simulink model "nine_bus_main_model"  (R2024a)
settings: Solver=FixedStepAuto  StartTime=0.0  StopTime=0.5  FixedStep=2e-5  MaxStep=1e-4  RelTol=1e-3
libraries: spsThreePhaseBreakerLib x18, spsThreePhaseVIMeasurementLib x18, simulink x18, sdolib x9, spsSeriesRLCBranchLib x9, spsThreePhasePISectionLineLib x6, spsThreePhaseSourceLib x3, spsThreePhaseParallelRLCLoadLib x3, spsThreePhaseTransformerTwoWindingsLib x3, spsThreePhaseFaultLib x2, spspowerguiLib x1
settings Model: Creator=Vaibhav Chaudhary  LastModifiedBy=Vaibhav Chaudhary

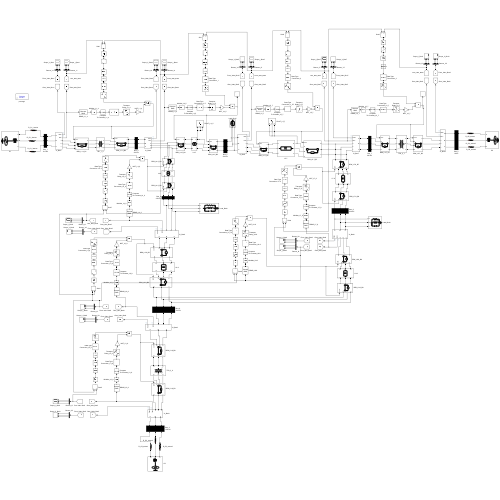
[thumbnail: Simulink's stored preview of the top-level diagram]
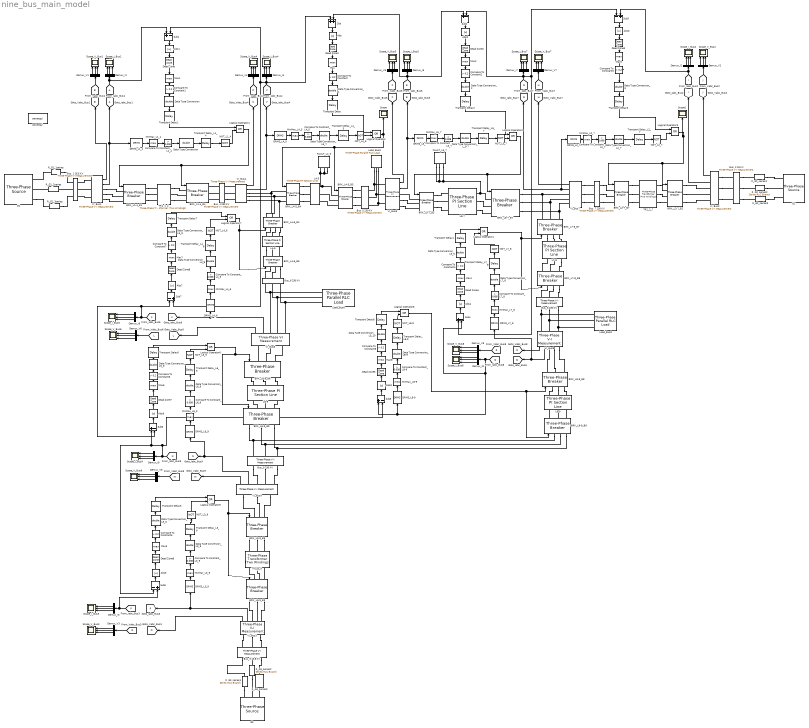
== system nine_bus_main_model ==
  Abs{,1..8} (9 alike) : Abs  SaturateOnIntegerOverflow=off
  "BRK_L1-4_B1 " : spsThreePhaseBreakerLib/Three-Phase Breaker  InitialState=closed  SwitchA=on  SwitchB=on  SwitchC=on  SwitchTimes="[1/60  5/60]"  External=on  BreakerResistance=0.01  SnubberResistance=1e6  SnubberCapacitance=inf  Measurements=None
  BRK_L1-4_B4 : spsThreePhaseBreakerLib/Three-Phase Breaker  InitialState=closed  SwitchA=on  SwitchB=on  SwitchC=on  SwitchTimes="[1/60  5/60]"  External=on  BreakerResistance=0.01  SnubberResistance=1e6  SnubberCapacitance=inf  Measurements=None
  "BRK_L2-7_B2 " : spsThreePhaseBreakerLib/Three-Phase Breaker  InitialState=closed  SwitchA=on  SwitchB=on  SwitchC=on  SwitchTimes="[1/60  5/60]"  External=on  BreakerResistance=0.01  SnubberResistance=1e6  SnubberCapacitance=inf  Measurements=None
  BRK_L2-7_B7 : spsThreePhaseBreakerLib/Three-Phase Breaker  InitialState=closed  SwitchA=on  SwitchB=on  SwitchC=on  SwitchTimes="[1/60  5/60]"  External=on  BreakerResistance=0.01  SnubberResistance=1e6  SnubberCapacitance=inf  Measurements=None
  "BRK_L3-9_B3 " : spsThreePhaseBreakerLib/Three-Phase Breaker  InitialState=closed  SwitchA=on  SwitchB=on  SwitchC=on  SwitchTimes="[1/60  5/60]"  External=on  BreakerResistance=0.01  SnubberResistance=1e6  SnubberCapacitance=inf  Measurements=None
  BRK_L3-9_B9 : spsThreePhaseBreakerLib/Three-Phase Breaker  InitialState=closed  SwitchA=on  SwitchB=on  SwitchC=on  SwitchTimes="[1/60  5/60]"  External=on  BreakerResistance=0.01  SnubberResistance=1e6  SnubberCapacitance=inf  Measurements=None
  BRK_L4-5_B4 : spsThreePhaseBreakerLib/Three-Phase Breaker  InitialState=closed  SwitchA=on  SwitchB=on  SwitchC=on  SwitchTimes="[1/60  5/60]"  External=on  BreakerResistance=0.01  SnubberResistance=1e6  SnubberCapacitance=inf  Measurements=None
  BRK_L4-5_B5 : spsThreePhaseBreakerLib/Three-Phase Breaker  InitialState=closed  SwitchA=on  SwitchB=on  SwitchC=on  SwitchTimes="[1/60  5/60]"  External=on  BreakerResistance=0.01  SnubberResistance=1e6  SnubberCapacitance=inf  Measurements=None
  BRK_L4-6_B4 : spsThreePhaseBreakerLib/Three-Phase Breaker  InitialState=closed  SwitchA=on  SwitchB=on  SwitchC=on  SwitchTimes="[1/60  5/60]"  External=on  BreakerResistance=0.01  SnubberResistance=1e6  SnubberCapacitance=inf  Measurements=None
  BRK_L4-6_B6 : spsThreePhaseBreakerLib/Three-Phase Breaker  InitialState=closed  SwitchA=on  SwitchB=on  SwitchC=on  SwitchTimes="[1/60  5/60]"  External=on  BreakerResistance=0.01  SnubberResistance=1e6  SnubberCapacitance=inf  Measurements=None
  BRK_L5-7_B5 : spsThreePhaseBreakerLib/Three-Phase Breaker  InitialState=closed  SwitchA=on  SwitchB=on  SwitchC=on  SwitchTimes="[1/60  5/60]"  External=on  BreakerResistance=0.01  SnubberResistance=1e6  SnubberCapacitance=inf  Measurements=None
  BRK_L5-7_B7 : spsThreePhaseBreakerLib/Three-Phase Breaker  InitialState=closed  SwitchA=on  SwitchB=on  SwitchC=on  SwitchTimes="[1/60  5/60]"  External=on  BreakerResistance=0.01  SnubberResistance=1e6  SnubberCapacitance=inf  Measurements=None
  BRK_L6-9_B6 : spsThreePhaseBreakerLib/Three-Phase Breaker  InitialState=closed  SwitchA=on  SwitchB=on  SwitchC=on  SwitchTimes="[1/60  5/60]"  External=on  BreakerResistance=0.01  SnubberResistance=1e6  SnubberCapacitance=inf  Measurements=None
  BRK_L6-9_B9 : spsThreePhaseBreakerLib/Three-Phase Breaker  InitialState=closed  SwitchA=on  SwitchB=on  SwitchC=on  SwitchTimes="[1/60  5/60]"  External=on  BreakerResistance=0.01  SnubberResistance=1e6  SnubberCapacitance=inf  Measurements=None
  BRK_L7-8_B7 : spsThreePhaseBreakerLib/Three-Phase Breaker  InitialState=closed  SwitchA=on  SwitchB=on  SwitchC=on  SwitchTimes="[1/60  5/60]"  External=on  BreakerResistance=0.01  SnubberResistance=1e6  SnubberCapacitance=inf  Measurements=None
  BRK_L7-8_B8 : spsThreePhaseBreakerLib/Three-Phase Breaker  InitialState=closed  SwitchA=on  SwitchB=on  SwitchC=on  SwitchTimes="[1/60  5/60]"  External=on  BreakerResistance=0.01  SnubberResistance=1e6  SnubberCapacitance=inf  Measurements=None
  BRK_L8-9_B8 : spsThreePhaseBreakerLib/Three-Phase Breaker  InitialState=closed  SwitchA=on  SwitchB=on  SwitchC=on  SwitchTimes="[1/60  5/60]"  External=on  BreakerResistance=0.01  SnubberResistance=1e6  SnubberCapacitance=inf  Measurements=None
  BRK_L8-9_B9 : spsThreePhaseBreakerLib/Three-Phase Breaker  InitialState=closed  SwitchA=on  SwitchB=on  SwitchC=on  SwitchTimes="[1/60  5/60]"  External=on  BreakerResistance=0.01  SnubberResistance=1e6  SnubberCapacitance=inf  Measurements=None
  Bus_1 16.5 KV : spsThreePhaseVIMeasurementLib/Three-Phase V-I Measurement  VoltageMeasurement=phase-to-phase  SetLabelV=on  LabelV=Vabc_B1  Vpu=on  VpuLL=off  CurrentMeasurement=yes  SetLabelI=on  LabelI=Iabc_B1  Ipu=on  Pbase=100e6  Vbase=16.5e3  OutputType=Complex  PhasorSimulation=off  PSBequivalent=0
  Bus_2 18 KV : spsThreePhaseVIMeasurementLib/Three-Phase V-I Measurement  VoltageMeasurement=phase-to-phase  SetLabelV=on  LabelV=Vabc_B2  Vpu=on  VpuLL=off  CurrentMeasurement=yes  SetLabelI=on  LabelI=Iabc_B2  Ipu=on  Pbase=100e6  Vbase=18e3  OutputType=Complex  PhasorSimulation=off  PSBequivalent=0
  Bus_3 13.8 KV : spsThreePhaseVIMeasurementLib/Three-Phase V-I Measurement  VoltageMeasurement=phase-to-phase  SetLabelV=on  LabelV=Vabc_B3  Vpu=on  VpuLL=off  CurrentMeasurement=yes  SetLabelI=on  LabelI=Iabc_B3  Ipu=on  Pbase=100e6  Vbase=13.8e3  OutputType=Complex  PhasorSimulation=off  PSBequivalent=0
  Bus_4 230 KV : spsThreePhaseVIMeasurementLib/Three-Phase V-I Measurement  VoltageMeasurement=phase-to-phase  SetLabelV=on  LabelV=Vabc_B4  Vpu=on  VpuLL=off  CurrentMeasurement=yes  SetLabelI=on  LabelI=Iabc_B4  Ipu=on  Pbase=100e6  Vbase=230e3  OutputType=Complex  PhasorSimulation=off  PSBequivalent=0
  Bus_5 230 KV : spsThreePhaseVIMeasurementLib/Three-Phase V-I Measurement  VoltageMeasurement=phase-to-phase  SetLabelV=on  LabelV=Vabc_B5  Vpu=on  VpuLL=off  CurrentMeasurement=yes  SetLabelI=on  LabelI=Iabc_B5  Ipu=on  Pbase=100e6  Vbase=230e3  OutputType=Complex  PhasorSimulation=off  PSBequivalent=0
  Bus_6 230 KV : spsThreePhaseVIMeasurementLib/Three-Phase V-I Measurement  VoltageMeasurement=phase-to-phase  SetLabelV=on  LabelV=Vabc_B6  Vpu=on  VpuLL=off  CurrentMeasurement=yes  SetLabelI=on  LabelI=Iabc_B6  Ipu=on  Pbase=100e6  Vbase=230e3  OutputType=Complex  PhasorSimulation=off  PSBequivalent=0
  Bus_7 230 KV : spsThreePhaseVIMeasurementLib/Three-Phase V-I Measurement  VoltageMeasurement=phase-to-phase  SetLabelV=on  LabelV=Vabc_B7  Vpu=on  VpuLL=off  CurrentMeasurement=yes  SetLabelI=on  LabelI=Iabc_B7  Ipu=on  Pbase=100e6  Vbase=230e3  OutputType=Complex  PhasorSimulation=off  PSBequivalent=0
  Bus_8 230 KV : spsThreePhaseVIMeasurementLib/Three-Phase V-I Measurement  VoltageMeasurement=phase-to-phase  SetLabelV=on  LabelV=Vabc_B8  Vpu=on  VpuLL=off  CurrentMeasurement=yes  SetLabelI=on  LabelI=Iabc_B8  Ipu=on  Pbase=100e6  Vbase=230e3  OutputType=Complex  PhasorSimulation=off  PSBequivalent=0
  Bus_9 230 KV : spsThreePhaseVIMeasurementLib/Three-Phase V-I Measurement  VoltageMeasurement=phase-to-phase  SetLabelV=on  LabelV=Vabc_B9  Vpu=on  VpuLL=off  CurrentMeasurement=yes  SetLabelI=on  LabelI=Iabc_B9  Ipu=on  Pbase=100e6  Vbase=230e3  OutputType=Complex  PhasorSimulation=off  PSBequivalent=0
  Compare To Constant{,1..8} (9 alike) : simulink/Logic and Bit Operations/Compare To Constant  relop=>  const=0.2  OutDataTypeStr=boolean
  Compare To Constant_L1_4 : simulink/Logic and Bit Operations/Compare To Constant  relop=>  const=0.008  OutDataTypeStr=boolean
  Compare To Constant_L2_7 : simulink/Logic and Bit Operations/Compare To Constant  relop=>  const=0.008  OutDataTypeStr=boolean
  Compare To Constant_L3_9 : simulink/Logic and Bit Operations/Compare To Constant  relop=>  const=0.008  OutDataTypeStr=boolean
  Compare To Constant_L4_5 : simulink/Logic and Bit Operations/Compare To Constant  relop=>  const=0.008  OutDataTypeStr=boolean
  Compare To Constant_L4_6 : simulink/Logic and Bit Operations/Compare To Constant  relop=>  const=0.008  OutDataTypeStr=boolean
  Compare To Constant_L5_7 : simulink/Logic and Bit Operations/Compare To Constant  relop=>  const=0.008  OutDataTypeStr=boolean
  Compare To Constant_L6_9 : simulink/Logic and Bit Operations/Compare To Constant  relop=>  const=0.008  OutDataTypeStr=boolean
  Compare To Constant_L7_8 : simulink/Logic and Bit Operations/Compare To Constant  relop=>  const=0.008  OutDataTypeStr=boolean
  Compare To Constant_L8-9 : simulink/Logic and Bit Operations/Compare To Constant  relop=>  const=0.008  OutDataTypeStr=boolean
  DRMS_L1_4 : sdolib/RMS Blocks/DRMS  Ts=1
  DRMS_L2_7 : sdolib/RMS Blocks/DRMS  Ts=1
  DRMS_L3_9 : sdolib/RMS Blocks/DRMS  Ts=1
  DRMS_L4_5 : sdolib/RMS Blocks/DRMS  Ts=1
  DRMS_L4_6 : sdolib/RMS Blocks/DRMS  Ts=1
  DRMS_L5_7 : sdolib/RMS Blocks/DRMS  Ts=1
  DRMS_L6_9 : sdolib/RMS Blocks/DRMS  Ts=1
  DRMS_L7_8 : sdolib/RMS Blocks/DRMS  Ts=1
  DRMS_L8-9 : sdolib/RMS Blocks/DRMS  Ts=1
  Data Type Conversion : DataTypeConversion  OutDataTypeStr=double  SaturateOnIntegerOverflow=off  RndMeth=Floor
  Data Type Conversion_1 : DataTypeConversion  OutDataTypeStr=double  SaturateOnIntegerOverflow=off  RndMeth=Floor
  Data Type Conversion_2 : DataTypeConversion  OutDataTypeStr=double  SaturateOnIntegerOverflow=off  RndMeth=Floor
  Data Type Conversion_3 : DataTypeConversion  OutDataTypeStr=double  SaturateOnIntegerOverflow=off  RndMeth=Floor
  Data Type Conversion_L5_{5..10} (6 alike) : DataTypeConversion  OutDataTypeStr=double  SaturateOnIntegerOverflow=off  RndMeth=Floor
  Data Type Conversion_L_5-7 : DataTypeConversion  OutDataTypeStr=double  SaturateOnIntegerOverflow=off  RndMeth=Floor
  Data Type Conversion_L2_7 : DataTypeConversion  OutDataTypeStr=double  SaturateOnIntegerOverflow=off  RndMeth=Floor
  Data Type Conversion_L3_9 : DataTypeConversion  OutDataTypeStr=double  SaturateOnIntegerOverflow=off  RndMeth=Floor
  Data Type Conversion_L4_6 : DataTypeConversion  OutDataTypeStr=double  SaturateOnIntegerOverflow=off  RndMeth=Floor
  Data Type Conversion_L6_9 : DataTypeConversion  OutDataTypeStr=double  SaturateOnIntegerOverflow=off  RndMeth=Floor
  Data Type Conversion_L7_8 : DataTypeConversion  OutDataTypeStr=double  SaturateOnIntegerOverflow=off  RndMeth=Floor
  Data Type Conversion_L8-9 : DataTypeConversion  OutDataTypeStr=double  SaturateOnIntegerOverflow=off  RndMeth=Floor
  Data Type Conversion : DataTypeConversion  OutDataTypeStr=double  SaturateOnIntegerOverflow=off  RndMeth=Floor
  Dead Zone{,2..8} (8 alike) : DeadZone  LowerValue=-0.01  UpperValue=0.01
  Dead Zone1 : DeadZone  LowerValue=0.01  UpperValue=inf
  Demux_I{1..9} (9 alike) : Demux  Outputs=3
  Demux_V{1..9} (9 alike) : Demux  Outputs=3
  FAULT_L4_5 : spsThreePhaseFaultLib/Three-Phase Fault  InitialStates=0  FaultA=on  FaultB=on  FaultC=on  GroundFault=on  SwitchTimes=[100 101]  External=off  SwitchStatus=NaN  FaultResistance=0.001  GroundResistance=0.001  SnubberResistance=1e6  SnubberCapacitance=inf  Measurements=None
  FAULT_L5_7 : spsThreePhaseFaultLib/Three-Phase Fault  InitialStates=0  FaultA=on  FaultB=on  FaultC=on  GroundFault=on  SwitchTimes=[0.05 0.1]  External=off  SwitchStatus=NaN  FaultResistance=0.001  GroundResistance=0.001  SnubberResistance=1e6  SnubberCapacitance=inf  Measurements=None
  From_Iabc_Bus1 : From  TagVisibility=global
  G1 : spsThreePhaseSourceLib/Three-Phase Source  InternalConnection=Yg  VoltagePhases=off  Voltage=16.5e3  PhaseAngle=0  Voltage_phases=[25e3 25e3 25e3]/sqrt(3)  PhaseAngles_phases=[0 -120 +120]  Frequency=50  NonIdealSource=on  SpecifyImpedance=off  Resistance=0  Inductance=0.1e-3  ShortCircuitLevel=100e6  BaseVoltage=16.5e3  XRratio=7  BusType=swing  Pref=10e3  Qref=0  Prefabc=[10e3, 10e3, 10e3]  Qrefabc=[0, 0, 0]  Qmin=-inf  Qmax=inf
  G2 : spsThreePhaseSourceLib/Three-Phase Source  InternalConnection=Yg  VoltagePhases=off  Voltage=18e3  PhaseAngle=0  Voltage_phases=[25e3 25e3 25e3]/sqrt(3)  PhaseAngles_phases=[0 -120 +120]  Frequency=50  NonIdealSource=on  SpecifyImpedance=off  Resistance=0  Inductance=0.15e-3  ShortCircuitLevel=100e6  BaseVoltage=18e3  XRratio=7  BusType=PV  Pref=163e3  Qref=0  Prefabc=[10e3, 10e3, 10e3]  Qrefabc=[0, 0, 0]  Qmin=-300e6  Qmax=300e6
  G3 : spsThreePhaseSourceLib/Three-Phase Source  InternalConnection=Yg  VoltagePhases=off  Voltage=13.8e3  PhaseAngle=0  Voltage_phases=[25e3 25e3 25e3]/sqrt(3)  PhaseAngles_phases=[0 -120 +120]  Frequency=50  NonIdealSource=on  SpecifyImpedance=off  Resistance=0  Inductance=0.2e-3  ShortCircuitLevel=100e6  BaseVoltage=13.8e3  XRratio=7  BusType=PV  Pref=85e3  Qref=0  Prefabc=[10e3, 10e3, 10e3]  Qrefabc=[0, 0, 0]  Qmin=-300e6  Qmax=300e6
  Goto_Iabc_Bus1 : Goto  TagVisibility=global
  L4-5 : spsThreePhasePISectionLineLib/Three-Phase PI Section Line  LConnTagsString=a|b|c  RConnTagsString=A|B|C  Length=100  Frequency=50  Resistances=[0.02 0.06]  Inductances=[1e-3 3e-3]  Capacitances=[2e-8 1e-8]
  L4-6 : spsThreePhasePISectionLineLib/Three-Phase PI Section Line  LConnTagsString=a|b|c  RConnTagsString=A|B|C  Length=100  Frequency=50  Resistances=[0.02 0.06]  Inductances=[1e-3 3e-3]  Capacitances=[2e-8 1e-8]
  L5-7 : spsThreePhasePISectionLineLib/Three-Phase PI Section Line  LConnTagsString=a|b|c  RConnTagsString=A|B|C  Length=100  Frequency=50  Resistances=[0.02 0.06]  Inductances=[1e-3 3e-3]  Capacitances=[2e-8 1e-8]
  L6-9 : spsThreePhasePISectionLineLib/Three-Phase PI Section Line  LConnTagsString=a|b|c  RConnTagsString=A|B|C  Length=100  Frequency=50  Resistances=[0.02 0.06]  Inductances=[1e-3 3e-3]  Capacitances=[2e-8 1e-8]
  L7-8 : spsThreePhasePISectionLineLib/Three-Phase PI Section Line  LConnTagsString=a|b|c  RConnTagsString=A|B|C  Length=100  Frequency=50  Resistances=[0.02 0.06]  Inductances=[1e-3 3e-3]  Capacitances=[2e-8 1e-8]
  L8-9 : spsThreePhasePISectionLineLib/Three-Phase PI Section Line  LConnTagsString=a|b|c  RConnTagsString=A|B|C  Length=100  Frequency=50  Resistances=[0.02 0.06]  Inductances=[1e-3 3e-3]  Capacitances=[2e-8 1e-8]
  Load_Bus5 : spsThreePhaseParallelRLCLoadLib/Three-Phase Parallel RLC Load  LConnTagsString=A|B|C  Configuration=Y (grounded)  NominalVoltage=230e3  Vabc=[1e3 1e3 1e3]  Vabcp=[1e3 1e3 1e3]  NominalFrequency=50  UnbalancedPower=off  ActivePower=125e6  InductivePower=50e6  CapacitivePower=50e6  Pabc=[10e3 9e3 11e3]  QLabc=[100 90 110]  QCabc=[100 90 110]  Pabcp=[10e3 9e3 11e3]  QLabcp=[100 90 110]  QCabcp=[100 90 110]  Measurements=None  LoadType=constant PQ
  Load_Bus6 : spsThreePhaseParallelRLCLoadLib/Three-Phase Parallel RLC Load  LConnTagsString=A|B|C  Configuration=Y (grounded)  NominalVoltage=230e3  Vabc=[1e3 1e3 1e3]  Vabcp=[1e3 1e3 1e3]  NominalFrequency=50  UnbalancedPower=off  ActivePower=90e6  InductivePower=30e6  CapacitivePower=30e6  Pabc=[10e3 9e3 11e3]  QLabc=[100 90 110]  QCabc=[100 90 110]  Pabcp=[10e3 9e3 11e3]  QLabcp=[100 90 110]  QCabcp=[100 90 110]  Measurements=None  LoadType=constant PQ
  Load_Bus8 : spsThreePhaseParallelRLCLoadLib/Three-Phase Parallel RLC Load  LConnTagsString=A|B|C  Configuration=Y (grounded)  NominalVoltage=230e3  Vabc=[1e3 1e3 1e3]  Vabcp=[1e3 1e3 1e3]  NominalFrequency=50  UnbalancedPower=off  ActivePower=100e6  InductivePower=35e6  CapacitivePower=35e6  Pabc=[10e3 9e3 11e3]  QLabc=[100 90 110]  QCabc=[100 90 110]  Pabcp=[10e3 9e3 11e3]  QLabcp=[100 90 110]  QCabcp=[100 90 110]  Measurements=None  LoadType=constant PQ
  Logical Operator{,1..8} (9 alike) : Logic  Operator=OR  AllPortsSameDT=off  OutDataTypeStr=boolean
  Max{,1..8} (9 alike) : MinMax  Function=max
  MinMax_L1_4 : MinMax  Function=max
  MinMax_L2_7 : MinMax  Function=max
  MinMax_L3_9 : MinMax  Function=max
  MinMax_L4_5 : MinMax  Function=max
  MinMax_L4_6 : MinMax  Function=max
  MinMax_L5_7 : MinMax  Function=max
  MinMax_L6_9 : MinMax  Function=max
  MinMax_L7_8 : MinMax  Function=max
  MinMax_L8-9 : MinMax  Function=max
  NOT_L1_4 : Logic  Operator=NOT  IconShape=distinctive  AllPortsSameDT=off  OutDataTypeStr=boolean
  NOT_L2_7 : Logic  Operator=NOT  IconShape=distinctive  AllPortsSameDT=off  OutDataTypeStr=boolean
  NOT_L3_9 : Logic  Operator=NOT  IconShape=distinctive  AllPortsSameDT=off  OutDataTypeStr=boolean
  NOT_L4_5 : Logic  Operator=NOT  IconShape=distinctive  AllPortsSameDT=off  OutDataTypeStr=boolean
  NOT_L4_6 : Logic  Operator=NOT  IconShape=distinctive  AllPortsSameDT=off  OutDataTypeStr=boolean
  NOT_L5_7 : Logic  Operator=NOT  IconShape=distinctive  AllPortsSameDT=off  OutDataTypeStr=boolean
  NOT_L6_9 : Logic  Operator=NOT  IconShape=distinctive  AllPortsSameDT=off  OutDataTypeStr=boolean
  NOT_L7_8 : Logic  Operator=NOT  IconShape=distinctive  AllPortsSameDT=off  OutDataTypeStr=boolean
  NOT_L8-9 : Logic  Operator=NOT  IconShape=distinctive  AllPortsSameDT=off  OutDataTypeStr=boolean
  R_G1_1series : spsSeriesRLCBranchLib/Series RLC Branch  LConnTagsString=__new0  RConnTagsString=__new0  BranchType=R  Resistance=0.01  Inductance=1e-3  SetiL0=off  InitialCurrent=0  Capacitance=1e-6  Setx0=off  InitialVoltage=0  Measurements=None
  R_G1_2series : spsSeriesRLCBranchLib/Series RLC Branch  LConnTagsString=__new0  RConnTagsString=__new0  BranchType=R  Resistance=0.01  Inductance=1e-3  SetiL0=off  InitialCurrent=0  Capacitance=1e-6  Setx0=off  InitialVoltage=0  Measurements=None
  R_G1_3series : spsSeriesRLCBranchLib/Series RLC Branch  LConnTagsString=__new0  RConnTagsString=__new0  BranchType=R  Resistance=0.01  Inductance=1e-3  SetiL0=off  InitialCurrent=0  Capacitance=1e-6  Setx0=off  InitialVoltage=0  Measurements=None
  R_G2_series1 : spsSeriesRLCBranchLib/Series RLC Branch  LConnTagsString=__new0  RConnTagsString=__new0  BranchType=R  Resistance=0.01  Inductance=1e-3  SetiL0=off  InitialCurrent=0  Capacitance=1e-6  Setx0=off  InitialVoltage=0  Measurements=None
  R_G2_series2 : spsSeriesRLCBranchLib/Series RLC Branch  LConnTagsString=__new0  RConnTagsString=__new0  BranchType=R  Resistance=0.01  Inductance=1e-3  SetiL0=off  InitialCurrent=0  Capacitance=1e-6  Setx0=off  InitialVoltage=0  Measurements=None
  R_G2_series3 : spsSeriesRLCBranchLib/Series RLC Branch  LConnTagsString=__new0  RConnTagsString=__new0  BranchType=R  Resistance=0.01  Inductance=1e-3  SetiL0=off  InitialCurrent=0  Capacitance=1e-6  Setx0=off  InitialVoltage=0  Measurements=None
  R_G3_series1 : spsSeriesRLCBranchLib/Series RLC Branch  LConnTagsString=__new0  RConnTagsString=__new0  BranchType=R  Resistance=0.01  Inductance=1e-3  SetiL0=off  InitialCurrent=0  Capacitance=1e-6  Setx0=off  InitialVoltage=0  Measurements=None
  R_G3_series2 : spsSeriesRLCBranchLib/Series RLC Branch  LConnTagsString=__new0  RConnTagsString=__new0  BranchType=R  Resistance=0.01  Inductance=1e-3  SetiL0=off  InitialCurrent=0  Capacitance=1e-6  Setx0=off  InitialVoltage=0  Measurements=None
  R_G3_series3 : spsSeriesRLCBranchLib/Series RLC Branch  LConnTagsString=__new0  RConnTagsString=__new0  BranchType=R  Resistance=0.01  Inductance=1e-3  SetiL0=off  InitialCurrent=0  Capacitance=1e-6  Setx0=off  InitialVoltage=0  Measurements=None
  Scope : Scope
  Scope1 : Scope
  Scope_I_Bus{1..9} (9 alike) : Scope  NumInputPorts=3
  Scope_V_Bus{1..9} (9 alike) : Scope  NumInputPorts=3
  Sub : Sum
  Sub{1..8} (8 alike) : Sum  Inputs=+-
  TR1_1_4 : spsThreePhaseTransformerTwoWindingsLib/Three-Phase Transformer (Two Windings)  Winding1Connection=Yg  Winding2Connection=Yg  CoreType=Three single-phase transformers  SetSaturation=off  Hysteresis=off  DataFile='hysteresis'  SetInitialFlux=off  Measurements=None  UNITS=pu  NominalPower=[ 100e6 , 50 ]  Winding1=[ 16.5e3 , 0.002 , 0.08 ]  Winding2=[ 230e3 , 0.002 , 0.08 ]  Rm=0.002  Lm=0.08  L0=0.5  Saturation=[ 0,0 ; 0.0024,1.2 ; 1.0,1.52 ]  InitialFluxes=[ 0.8 , -0.8 , 0.7 ]  BreakLoop=off  DiscreteSolver=Trapezoidal iterative  DataType=off  TransfoNumber=1
  TR2_2_7 : spsThreePhaseTransformerTwoWindingsLib/Three-Phase Transformer (Two Windings)  Winding1Connection=Yg  Winding2Connection=Yg  CoreType=Three single-phase transformers  SetSaturation=off  Hysteresis=off  DataFile='hysteresis'  SetInitialFlux=off  Measurements=None  UNITS=pu  NominalPower=[ 100e6 , 50]  Winding1=[ 18e3 , 0.002 , 0.08 ]  Winding2=[ 23e3 , 0.002 , 0.08 ]  Rm=0.002  Lm=0.08  L0=0.5  Saturation=[ 0,0 ; 0.0024,1.2 ; 1.0,1.52 ]  InitialFluxes=[ 0.8 , -0.8 , 0.7 ]  BreakLoop=off  DiscreteSolver=Trapezoidal iterative  DataType=off  TransfoNumber=1
  TR3_3_9 : spsThreePhaseTransformerTwoWindingsLib/Three-Phase Transformer (Two Windings)  Winding1Connection=Yg  Winding2Connection=Yg  CoreType=Three single-phase transformers  SetSaturation=off  Hysteresis=off  DataFile='hysteresis'  SetInitialFlux=off  Measurements=None  UNITS=pu  NominalPower=[ 100e6 , 50 ]  Winding1=[ 16.5e3 , 0.002 , 0.08 ]  Winding2=[ 230e3 , 0.002 , 0.08 ]  Rm=0.002  Lm=0.08  L0=0.5  Saturation=[ 0,0 ; 0.0024,1.2 ; 1.0,1.52 ]  InitialFluxes=[ 0.8 , -0.8 , 0.7 ]  BreakLoop=off  DiscreteSolver=Trapezoidal iterative  DataType=off  TransfoNumber=1
  Transport Delay{,1..8} (9 alike) : TransportDelay  DelayTime=0.005
  Transport Delay_L1_4 : TransportDelay  DelayTime=0.02
  Transport Delay_L2_7 : TransportDelay  DelayTime=0.02
  Transport Delay_L3_9 : TransportDelay  DelayTime=0.02
  Transport Delay_L4_5 : TransportDelay  DelayTime=0.02
  Transport Delay_L4_6 : TransportDelay  DelayTime=0.02
  Transport Delay_L5_7 : TransportDelay  DelayTime=0.02
  Transport Delay_L6_9 : TransportDelay  DelayTime=0.02
  Transport Delay_L7_8 : TransportDelay  DelayTime=0.02
  Transport Delay_L8-9 : TransportDelay  DelayTime=0.02
  VI_Bus1 : spsThreePhaseVIMeasurementLib/Three-Phase V-I Measurement  VoltageMeasurement=phase-to-phase  SetLabelV=off  LabelV=Vabc  Vpu=off  VpuLL=on  CurrentMeasurement=yes  SetLabelI=off  LabelI=Iabc  Ipu=on  Pbase=100e6  Vbase=16.5e3  OutputType=Complex  PhasorSimulation=off  PSBequivalent=0
  VI_Bus2 : spsThreePhaseVIMeasurementLib/Three-Phase V-I Measurement  VoltageMeasurement=phase-to-phase  SetLabelV=off  LabelV=Vabc  Vpu=off  VpuLL=on  CurrentMeasurement=yes  SetLabelI=off  LabelI=Iabc  Ipu=on  Pbase=100e6  Vbase=18e3  OutputType=Complex  PhasorSimulation=off  PSBequivalent=0
  VI_Bus3 : spsThreePhaseVIMeasurementLib/Three-Phase V-I Measurement  VoltageMeasurement=phase-to-phase  SetLabelV=off  LabelV=Vabc  Vpu=on  VpuLL=off  CurrentMeasurement=yes  SetLabelI=off  LabelI=Iabc  Ipu=on  Pbase=100e6  Vbase=13.8e3  OutputType=Complex  PhasorSimulation=off  PSBequivalent=0
  VI_Bus{4..6,9} (4 alike) : spsThreePhaseVIMeasurementLib/Three-Phase V-I Measurement  VoltageMeasurement=phase-to-phase  SetLabelV=off  LabelV=Vabc  Vpu=off  VpuLL=on  CurrentMeasurement=yes  SetLabelI=off  LabelI=Iabc  Ipu=on  Pbase=100e6  Vbase=250e3  OutputType=Complex  PhasorSimulation=off  PSBequivalent=0
  VI_Bus7 : spsThreePhaseVIMeasurementLib/Three-Phase V-I Measurement  VoltageMeasurement=phase-to-phase  SetLabelV=off  LabelV=Vabc  Vpu=off  VpuLL=off  CurrentMeasurement=yes  SetLabelI=off  LabelI=Iabc  Ipu=on  Pbase=100e6  Vbase=250e3  OutputType=Complex  PhasorSimulation=off  PSBequivalent=0
  VI_Bus8 : spsThreePhaseVIMeasurementLib/Three-Phase V-I Measurement  VoltageMeasurement=phase-to-phase  SetLabelV=off  LabelV=Vabc  Vpu=off  VpuLL=off  CurrentMeasurement=yes  SetLabelI=off  LabelI=Iabc  Ipu=on  Pbase=100e6  Vbase=250e3  OutputType=Complex  PhasorSimulation=off  PSBequivalent=0
  powergui : spspowerguiLib/powergui  Priority=1  SimulationMode=Discrete  SampleTime=2e-5  frequency=60  Iterations=50  frequencyindice=0  Pbase=100e6  ErrMax=1e-4  UnitsV=kV  UnitsW=MW  buscounter=0  FunctionMessages=off  echomessages=off  EnableUseOfTLC=off  CurrentSourceSwitches=off  DisableSnubberDevices=off  DisableRonSwitches=off  DisableVfSwitches=off  DisplayEquations=off  AutomaticDiscreteSolvers=off  SolverType=Tustin/Backward Euler (TBE)  Interpol=off  ExternalGateDelay=off  methode=off  Ts=100  x0status=blocks  SPID=on  SwTol=0  HookPort=off  NonlinearTolerance=1e-4  nMaxIteration=100  ContinueOnMaxIteration=off  RestoreLinks=warning  ResistiveCurrentMeasurement=off  Frange=[0:2:500]  Ylog=off  Xlog=on  ShowGrid=off  save=off  variable=ZData  structure=0  ZoomFFT=off  StartTime=0.0  cycles=1  DisplayStyle=1  fundamental=60  FreqAxis=off  MaxFrequency=1000  frequencyindicesteady=1  RmsSteady=1  display=off
  tag scope: B=global, C=global, E=global, F=global, G=global, H=global, I=global, J=global, K=global, L=global, M=global, N=global, O=global, P=global, Q=global, R=global, V=global
  wires:
  Demux_V1/1 -> Scope_V_Bus1/1
  Demux_I1/1 -> Scope_I_Bus1/1
  Demux_I1/2 -> Scope_I_Bus1/2
  Demux_I1/3 -> Scope_I_Bus1/3
  VI_Bus1/1 -> [B]
  Demux_V4/2 -> Scope_V_Bus4/2
  VI_Bus4/1 -> [C]
  Demux_V4/3 -> Scope_V_Bus4/3
  [C] -> Demux_V4/1
  Demux_V4/1 -> Scope_V_Bus4/1
  VI_Bus5/1 -> [F]
  Demux_I5/2 -> Scope_I_Bus5/2
  Demux_V5/3 -> Scope_V_Bus5/3
  Demux_I5/3 -> Scope_I_Bus5/3
  Demux_V5/1 -> Scope_V_Bus5/1
  Demux_V5/2 -> Scope_V_Bus5/2
  Demux_I5/1 -> Scope_I_Bus5/1
  [E] -> Demux_I5/1, Sub2/1, Sub/2
  VI_Bus7/1 -> [H]
  Demux_V7/3 -> Scope_V_Bus7/3
  Demux_I7/3 -> Scope_I_Bus7/3
  Demux_I7/2 -> Scope_I_Bus7/2
  Demux_I7/1 -> Scope_I_Bus7/1
  Demux_V7/1 -> Scope_V_Bus7/1
  [H] -> Demux_V7/1
  Demux_V7/2 -> Scope_V_Bus7/2
  VI_Bus2/2 -> [I]
  Demux_V2/1 -> Scope_V_Bus2/1
  Demux_I2/1 -> Scope_I_Bus2/1
  Demux_V2/2 -> Scope_V_Bus2/2
  [J] -> Demux_V2/1
  Demux_I2/2 -> Scope_I_Bus2/2
  VI_Bus2/1 -> [J]
  Demux_V2/3 -> Scope_V_Bus2/3
  Demux_I2/3 -> Scope_I_Bus2/3
  [K] -> Sub6/2, Sub7/2, Demux_I6/1
  Demux_I6/1 -> Scope_I_Bus6/1
  Demux_V6/2 -> Scope_V_Bus6/2
  VI_Bus6/1 -> [L]
  Demux_I6/3 -> Scope_I_Bus6/3
  Demux_V6/3 -> Scope_V_Bus6/3
  [L] -> Demux_V6/1
  Demux_V6/1 -> Scope_V_Bus6/1
  Demux_I6/2 -> Scope_I_Bus6/2
  [M] -> Demux_V9/1
  Demux_I9/1 -> Scope_I_Bus9/1
  Demux_I9/2 -> Scope_I_Bus9/2
  Demux_V9/2 -> Scope_V_Bus9/2
  VI_Bus9/2 -> DRMS_L6_9/1, [N]
  Demux_V9/3 -> Scope_V_Bus9/3
  Demux_I9/3 -> Scope_I_Bus9/3
  Demux_V9/1 -> Scope_V_Bus9/1
  VI_Bus9/1 -> [M]
  [O] -> Demux_V3/1
  [P] -> Sub5/1, Demux_I3/1
  Demux_I3/1 -> Scope_I_Bus3/1
  Demux_I3/2 -> Scope_I_Bus3/2
  Demux_V3/2 -> Scope_V_Bus3/2
  VI_Bus3/2 -> [P], DRMS_L3_9/1
  Demux_V3/3 -> Scope_V_Bus3/3
  Demux_I3/3 -> Scope_I_Bus3/3
  Demux_V3/1 -> Scope_V_Bus3/1
  VI_Bus3/1 -> [O]
  [R] -> Demux_V8/1
  [Q] -> Demux_I8/1, Sub4/2, Sub8/1, DRMS_L8-9/1
  Demux_I8/1 -> Scope_I_Bus8/1
  Demux_I8/2 -> Scope_I_Bus8/2
  Demux_V8/2 -> Scope_V_Bus8/2
  VI_Bus8/2 -> DRMS_L7_8/1, [Q]
  Demux_V8/3 -> Scope_V_Bus8/3
  Demux_I8/3 -> Scope_I_Bus8/3
  Demux_V8/1 -> Scope_V_Bus8/1
  VI_Bus8/1 -> [R]
  Transport Delay_L6_9/1 -> NOT_L6_9/1
  Demux_I4/1 -> Scope_I_Bus4/1
  Demux_I4/3 -> Scope_I_Bus4/3
  Demux_I4/2 -> Scope_I_Bus4/2
  Transport Delay_L5_7/1 -> NOT_L5_7/1
  Transport Delay_L2_7/1 -> NOT_L2_7/1
  Transport Delay_L4_6/1 -> NOT_L4_6/1
  VI_Bus6/2 -> [K], DRMS_L4_6/1
  DRMS_L1_4/1 -> MinMax_L1_4/1
  MinMax_L1_4/1 -> Compare To Constant_L1_4/1
  Transport Delay_L1_4/1 -> NOT_L1_4/1
  DRMS_L4_5/1 -> MinMax_L4_5/1
  MinMax_L4_5/1 -> Compare To Constant_L4_5/1
  Compare To Constant_L1_4/1 -> Data Type Conversion/1
  Data Type Conversion/1 -> Transport Delay_L1_4/1
  Compare To Constant_L4_5/1 -> Data Type Conversion_L5_7/1
  Data Type Conversion_L5_7/1 -> Transport Delay_L4_5/1
  VI_Bus5/2 -> [E], DRMS_L5_7/1
  MinMax_L5_7/1 -> Compare To Constant_L5_7/1
  Data Type Conversion_L_5-7/1 -> Transport Delay_L5_7/1
  Compare To Constant_L5_7/1 -> Data Type Conversion_L_5-7/1
  DRMS_L5_7/1 -> MinMax_L5_7/1
  Data Type Conversion_L2_7/1 -> Transport Delay_L2_7/1
  Compare To Constant_L2_7/1 -> Data Type Conversion_L2_7/1
  DRMS_L2_7/1 -> MinMax_L2_7/1
  VI_Bus7/2 -> [G], DRMS_L2_7/1
  MinMax_L2_7/1 -> Compare To Constant_L2_7/1
  Data Type Conversion_L7_8/1 -> Transport Delay_L7_8/1
  MinMax_L7_8/1 -> Compare To Constant_L7_8/1
  DRMS_L7_8/1 -> MinMax_L7_8/1
  Compare To Constant_L7_8/1 -> Data Type Conversion_L7_8/1
  Transport Delay_L7_8/1 -> NOT_L7_8/1
  MinMax_L3_9/1 -> Compare To Constant_L3_9/1
  DRMS_L3_9/1 -> MinMax_L3_9/1
  Compare To Constant_L3_9/1 -> Data Type Conversion_L3_9/1
  Data Type Conversion_L3_9/1 -> Transport Delay_L3_9/1
  Transport Delay_L3_9/1 -> NOT_L3_9/1
  MinMax_L6_9/1 -> Compare To Constant_L6_9/1
  DRMS_L6_9/1 -> MinMax_L6_9/1
  Compare To Constant_L6_9/1 -> Data Type Conversion_L6_9/1
  Data Type Conversion_L6_9/1 -> Transport Delay_L6_9/1
  Compare To Constant_L4_6/1 -> Data Type Conversion_L4_6/1
  MinMax_L4_6/1 -> Compare To Constant_L4_6/1
  DRMS_L4_6/1 -> MinMax_L4_6/1
  Data Type Conversion_L4_6/1 -> Transport Delay_L4_6/1
  Sub/1 -> Abs/1
  Abs/1 -> Dead Zone1/1
  [F] -> Demux_V5/1
  Max/1 -> Compare To Constant/1
  Compare To Constant/1 -> Data Type Conversion_1/1
  Data Type Conversion_1/1 -> Transport Delay/1
  Transport Delay/1 -> Logical Operator/1
  Data Type Conversion/1 -> Transport Delay1/1
  Abs1/1 -> Dead Zone/1
  Compare To Constant1/1 -> Data Type Conversion/1
  Sub1/1 -> Abs1/1
  Max1/1 -> Compare To Constant1/1
  Transport Delay1/1 -> Logical Operator1/1
  VI_Bus1/2 -> Goto_Iabc_Bus1/1, DRMS_L1_4/1
  NOT_L1_4/1 -> Logical Operator1/2
  Logical Operator1/1 -> "BRK_L1-4_B1 "/1, BRK_L1-4_B4/1
  Data Type Conversion_2/1 -> Transport Delay2/1
  Transport Delay2/1 -> Logical Operator2/1
  Compare To Constant2/1 -> Data Type Conversion_2/1
  Max2/1 -> Compare To Constant2/1
  NOT_L5_7/1 -> Logical Operator2/2
  Logical Operator2/1 -> BRK_L5-7_B5/1, BRK_L5-7_B7/1
  NOT_L2_7/1 -> Logical Operator3/2
  Logical Operator3/1 -> Scope1/1, "BRK_L2-7_B2 "/1, BRK_L2-7_B7/1
  Data Type Conversion_3/1 -> Transport Delay3/1
  Abs3/1 -> Dead Zone3/1
  Compare To Constant3/1 -> Data Type Conversion_3/1
  Sub3/1 -> Abs3/1
  Max3/1 -> Compare To Constant3/1
  [G] -> Sub3/2, Sub4/1, Sub2/2, Demux_I7/1
  Data Type Conversion_L5_5/1 -> Transport Delay4/1
  Compare To Constant4/1 -> Data Type Conversion_L5_5/1
  Sub4/1 -> Abs4/1
  Max4/1 -> Compare To Constant4/1
  Transport Delay3/1 -> Logical Operator3/1
  Transport Delay4/1 -> Logical Operator4/1
  NOT_L7_8/1 -> Logical Operator4/2
  Logical Operator4/1 -> BRK_L7-8_B8/1, BRK_L7-8_B7/1
  Sub5/1 -> Abs5/1
  Compare To Constant5/1 -> Data Type Conversion_L5_6/1
  Data Type Conversion_L5_6/1 -> Transport Delay5/1
  Abs5/1 -> Dead Zone6/1
  Max5/1 -> Compare To Constant5/1
  NOT_L3_9/1 -> Logical Operator5/2
  Transport Delay5/1 -> Logical Operator5/1
  Logical Operator5/1 -> "BRK_L3-9_B3 "/1, BRK_L3-9_B9/1
  NOT_L6_9/1 -> Logical Operator6/2
  Logical Operator6/1 -> BRK_L6-9_B9/1, BRK_L6-9_B6/1
  Sub6/1 -> Abs6/1
  Compare To Constant6/1 -> Data Type Conversion_L5_8/1
  Data Type Conversion_L5_8/1 -> Transport Delay6/1
  Max6/1 -> Compare To Constant6/1
  Transport Delay6/1 -> Logical Operator6/1
  Max7/1 -> Compare To Constant7/1
  Data Type Conversion_L5_9/1 -> Transport Delay7/1
  Sub7/1 -> Abs7/1
  Compare To Constant7/1 -> Data Type Conversion_L5_9/1
  Transport Delay7/1 -> Logical Operator7/1
  Abs7/1 -> Dead Zone8/1
  NOT_L4_6/1 -> Logical Operator7/2
  Logical Operator7/1 -> BRK_L4-6_B6/1, BRK_L4-6_B4/1
  NOT_L8-9/1 -> Logical Operator8/2
  Transport Delay8/1 -> Logical Operator8/1
  Logical Operator8/1 -> BRK_L8-9_B8/1, BRK_L8-9_B9/1
  Compare To Constant8/1 -> Data Type Conversion_L5_10/1
  Data Type Conversion_L5_10/1 -> Transport Delay8/1
  Abs8/1 -> Dead Zone5/1
  Max8/1 -> Compare To Constant8/1
  Transport Delay_L8-9/1 -> NOT_L8-9/1
  MinMax_L8-9/1 -> Compare To Constant_L8-9/1
  Sub8/1 -> Abs8/1
  DRMS_L8-9/1 -> MinMax_L8-9/1
  Compare To Constant_L8-9/1 -> Data Type Conversion_L8-9/1
  Data Type Conversion_L8-9/1 -> Transport Delay_L8-9/1
  Dead Zone/1 -> Max1/1
  Dead Zone1/1 -> Max/1
  Dead Zone2/1 -> Max2/1
  Sub2/1 -> Abs2/1
  Dead Zone3/1 -> Max3/1
  Dead Zone4/1 -> Max4/1
  Dead Zone5/1 -> Max8/1
  Dead Zone6/1 -> Max5/1
  Dead Zone7/1 -> Max6/1
  Dead Zone8/1 -> Max7/1
  Logical Operator/1 -> BRK_L4-5_B4/1, BRK_L4-5_B5/1, Scope/1
  Transport Delay_L4_5/1 -> NOT_L4_5/1
  NOT_L4_5/1 -> Logical Operator/2
  VI_Bus4/2 -> DRMS_L4_5/1, [V]
  [B] -> Demux_V1/1
  From_Iabc_Bus1/1 -> Sub1/1, Demux_I1/1
  Abs2/1 -> Dead Zone2/1
  [I] -> Sub3/1, Demux_I2/1
  Abs4/1 -> Dead Zone4/1
  [N] -> Sub8/2, Sub5/2, Sub6/1, Demux_I9/1
  Abs6/1 -> Dead Zone7/1
  [V] -> Sub/1, Sub1/2, Sub7/1, Demux_I4/1
  Demux_V1/3 -> Scope_V_Bus1/3
  Demux_V1/2 -> Scope_V_Bus1/2
  connections:
  VI_Bus1/LConn3 -- Bus_1 16.5 KV/LConn3
  VI_Bus1/LConn2 -- Bus_1 16.5 KV/LConn2
  VI_Bus1/LConn1 -- Bus_1 16.5 KV/LConn1
  VI_Bus5/LConn3 -- Bus_5 230 KV/LConn3 -- Load_Bus5/LConn3
  VI_Bus5/LConn2 -- Bus_5 230 KV/LConn2 -- Load_Bus5/LConn2
  VI_Bus5/LConn1 -- Bus_5 230 KV/LConn1 -- Load_Bus5/LConn1
  VI_Bus2/LConn2 -- Bus_2 18 KV/LConn2
  VI_Bus2/LConn1 -- Bus_2 18 KV/LConn1
  VI_Bus2/LConn3 -- Bus_2 18 KV/LConn3
  VI_Bus7/LConn1 -- Bus_7 230 KV/LConn1
  VI_Bus7/LConn2 -- Bus_7 230 KV/LConn2
  VI_Bus7/LConn3 -- Bus_7 230 KV/LConn3
  Bus_8 230 KV/LConn3 -- VI_Bus8/LConn3 -- Load_Bus8/LConn3
  Bus_8 230 KV/LConn2 -- VI_Bus8/LConn2 -- Load_Bus8/LConn2
  Bus_8 230 KV/LConn1 -- VI_Bus8/LConn1 -- Load_Bus8/LConn1
  VI_Bus3/LConn1 -- Bus_3 13.8 KV/LConn1
  VI_Bus3/LConn2 -- Bus_3 13.8 KV/LConn2
  VI_Bus3/LConn3 -- Bus_3 13.8 KV/LConn3
  "BRK_L3-9_B3 "/LConn3 -- TR3_3_9/LConn3
  "BRK_L3-9_B3 "/LConn2 -- TR3_3_9/LConn2
  "BRK_L3-9_B3 "/LConn1 -- TR3_3_9/LConn1
  TR1_1_4/RConn1 -- BRK_L1-4_B4/LConn1
  BRK_L1-4_B4/LConn2 -- TR1_1_4/RConn2
  TR1_1_4/RConn3 -- BRK_L1-4_B4/LConn3
  "BRK_L1-4_B1 "/RConn1 -- TR1_1_4/LConn1
  "BRK_L1-4_B1 "/RConn2 -- TR1_1_4/LConn2
  "BRK_L1-4_B1 "/RConn3 -- TR1_1_4/LConn3
  "BRK_L2-7_B2 "/RConn1 -- VI_Bus2/RConn1
  "BRK_L2-7_B2 "/RConn2 -- VI_Bus2/RConn2
  "BRK_L2-7_B2 "/RConn3 -- VI_Bus2/RConn3
  R_G1_1series/LConn1 -- G1/RConn1
  R_G1_2series/LConn1 -- G1/RConn2
  G1/RConn3 -- R_G1_3series/LConn1
  R_G1_1series/RConn1 -- Bus_1 16.5 KV/RConn1
  R_G1_3series/RConn1 -- Bus_1 16.5 KV/RConn3
  Bus_1 16.5 KV/RConn2 -- R_G1_2series/RConn1
  VI_Bus1/RConn1 -- "BRK_L1-4_B1 "/LConn1
  VI_Bus1/RConn2 -- "BRK_L1-4_B1 "/LConn2
  VI_Bus1/RConn3 -- "BRK_L1-4_B1 "/LConn3
  Bus_4 230 KV/RConn1 -- BRK_L1-4_B4/RConn1
  Bus_4 230 KV/RConn2 -- BRK_L1-4_B4/RConn2
  Bus_4 230 KV/RConn3 -- BRK_L1-4_B4/RConn3
  VI_Bus4/LConn1 -- Bus_4 230 KV/LConn1
  VI_Bus4/LConn2 -- Bus_4 230 KV/LConn2
  Bus_4 230 KV/LConn3 -- VI_Bus4/LConn3
  BRK_L4-6_B4/LConn2 -- L4-6/LConn2
  BRK_L4-6_B4/LConn3 -- L4-6/LConn3
  BRK_L4-6_B4/LConn1 -- L4-6/LConn1
  VI_Bus4/RConn1 -- BRK_L4-6_B4/RConn1 -- BRK_L4-5_B4/LConn1
  VI_Bus4/RConn2 -- BRK_L4-6_B4/RConn2 -- BRK_L4-5_B4/LConn2
  VI_Bus4/RConn3 -- BRK_L4-6_B4/RConn3 -- BRK_L4-5_B4/LConn3
  BRK_L4-6_B6/RConn3 -- L4-6/RConn3
  BRK_L4-6_B6/RConn2 -- L4-6/RConn2
  L4-6/RConn1 -- BRK_L4-6_B6/RConn1
  BRK_L4-5_B4/RConn3 -- L4-5/LConn3
  BRK_L4-5_B4/RConn2 -- L4-5/LConn2
  BRK_L4-5_B5/LConn3 -- L4-5/RConn3
  BRK_L4-5_B5/LConn2 -- L4-5/RConn2
  BRK_L4-5_B5/LConn1 -- FAULT_L4_5/LConn3 -- FAULT_L4_5/LConn2 -- FAULT_L4_5/LConn1 -- L4-5/RConn1
  BRK_L4-5_B5/RConn1 -- Bus_5 230 KV/RConn1
  BRK_L4-5_B5/RConn2 -- Bus_5 230 KV/RConn2
  BRK_L4-5_B5/RConn3 -- Bus_5 230 KV/RConn3
  BRK_L5-7_B5/LConn1 -- VI_Bus5/RConn1
  VI_Bus5/RConn3 -- BRK_L5-7_B5/LConn3
  VI_Bus5/RConn2 -- BRK_L5-7_B5/LConn2
  BRK_L5-7_B5/RConn1 -- L5-7/LConn1
  BRK_L5-7_B5/RConn2 -- L5-7/LConn2
  BRK_L5-7_B5/RConn3 -- L5-7/LConn3
  BRK_L5-7_B7/LConn1 -- FAULT_L5_7/LConn3 -- FAULT_L5_7/LConn2 -- FAULT_L5_7/LConn1 -- L5-7/RConn1
  L5-7/RConn2 -- BRK_L5-7_B7/LConn2
  L5-7/RConn3 -- BRK_L5-7_B7/LConn3
  Bus_6 230 KV/RConn2 -- BRK_L4-6_B6/LConn2
  BRK_L4-6_B6/LConn3 -- Bus_6 230 KV/RConn3
  BRK_L4-6_B6/LConn1 -- Bus_6 230 KV/RConn1
  VI_Bus6/RConn1 -- Bus_6 230 KV/LConn1 -- Load_Bus6/LConn1
  VI_Bus6/RConn2 -- Bus_6 230 KV/LConn2 -- Load_Bus6/LConn2
  VI_Bus6/RConn3 -- Bus_6 230 KV/LConn3 -- Load_Bus6/LConn3
  BRK_L6-9_B6/LConn2 -- VI_Bus6/LConn2
  BRK_L6-9_B6/LConn3 -- VI_Bus6/LConn3
  BRK_L6-9_B6/LConn1 -- VI_Bus6/LConn1
  BRK_L6-9_B6/RConn2 -- L6-9/LConn2
  BRK_L6-9_B6/RConn3 -- L6-9/LConn3
  BRK_L6-9_B6/RConn1 -- L6-9/LConn1
  BRK_L6-9_B9/LConn2 -- L6-9/RConn2
  BRK_L6-9_B9/LConn3 -- L6-9/RConn3
  BRK_L6-9_B9/LConn1 -- L6-9/RConn1
  BRK_L6-9_B9/RConn3 -- BRK_L8-9_B9/LConn3 -- Bus_9 230 KV/LConn3
  BRK_L6-9_B9/RConn2 -- BRK_L8-9_B9/LConn2 -- Bus_9 230 KV/LConn2
  BRK_L6-9_B9/RConn1 -- BRK_L8-9_B9/LConn1 -- Bus_9 230 KV/LConn1
  Bus_9 230 KV/RConn3 -- VI_Bus9/RConn3
  Bus_9 230 KV/RConn2 -- VI_Bus9/RConn2
  Bus_9 230 KV/RConn1 -- VI_Bus9/RConn1
  R_G2_series1/RConn1 -- G2/RConn1
  R_G2_series2/RConn1 -- G2/RConn2
  R_G2_series3/RConn1 -- G2/RConn3
  Bus_2 18 KV/RConn3 -- R_G2_series3/LConn1
  Bus_2 18 KV/RConn2 -- R_G2_series2/LConn1
  Bus_2 18 KV/RConn1 -- R_G2_series1/LConn1
  TR2_2_7/LConn2 -- "BRK_L2-7_B2 "/LConn2
  TR2_2_7/LConn3 -- "BRK_L2-7_B2 "/LConn3
  TR2_2_7/LConn1 -- "BRK_L2-7_B2 "/LConn1
  BRK_L2-7_B7/RConn3 -- TR2_2_7/RConn3
  BRK_L2-7_B7/RConn2 -- TR2_2_7/RConn2
  Bus_7 230 KV/RConn3 -- BRK_L2-7_B7/LConn3
  Bus_7 230 KV/RConn2 -- BRK_L2-7_B7/LConn2
  Bus_7 230 KV/RConn1 -- BRK_L2-7_B7/LConn1
  BRK_L5-7_B7/RConn1 -- BRK_L7-8_B7/RConn1 -- VI_Bus7/RConn1
  BRK_L5-7_B7/RConn2 -- BRK_L7-8_B7/RConn2 -- VI_Bus7/RConn2
  BRK_L5-7_B7/RConn3 -- BRK_L7-8_B7/RConn3 -- VI_Bus7/RConn3
  BRK_L7-8_B7/LConn2 -- L7-8/LConn2
  BRK_L7-8_B7/LConn3 -- L7-8/LConn3
  BRK_L7-8_B7/LConn1 -- L7-8/LConn1
  BRK_L7-8_B8/RConn2 -- L7-8/RConn2
  BRK_L7-8_B8/RConn1 -- L7-8/RConn1
  BRK_L7-8_B8/LConn2 -- Bus_8 230 KV/RConn2
  BRK_L7-8_B8/LConn3 -- Bus_8 230 KV/RConn3
  BRK_L7-8_B8/LConn1 -- Bus_8 230 KV/RConn1
  BRK_L8-9_B8/LConn3 -- L8-9/LConn3
  BRK_L8-9_B8/LConn2 -- L8-9/LConn2
  BRK_L8-9_B8/LConn1 -- L8-9/LConn1
  VI_Bus8/RConn3 -- BRK_L8-9_B8/RConn3
  VI_Bus8/RConn2 -- BRK_L8-9_B8/RConn2
  BRK_L8-9_B8/RConn1 -- VI_Bus8/RConn1
  L7-8/RConn3 -- BRK_L7-8_B8/RConn3
  BRK_L8-9_B9/RConn3 -- L8-9/RConn3
  BRK_L8-9_B9/RConn2 -- L8-9/RConn2
  BRK_L8-9_B9/RConn1 -- L8-9/RConn1
  R_G3_series3/LConn1 -- G3/RConn3
  R_G3_series2/LConn1 -- G3/RConn2
  R_G3_series1/LConn1 -- G3/RConn1
  Bus_3 13.8 KV/RConn3 -- R_G3_series3/RConn1
  Bus_3 13.8 KV/RConn2 -- R_G3_series2/RConn1
  Bus_3 13.8 KV/RConn1 -- R_G3_series1/RConn1
  "BRK_L3-9_B3 "/RConn3 -- VI_Bus3/RConn3
  "BRK_L3-9_B3 "/RConn2 -- VI_Bus3/RConn2
  "BRK_L3-9_B3 "/RConn1 -- VI_Bus3/RConn1
  BRK_L3-9_B9/RConn1 -- TR3_3_9/RConn1
  BRK_L3-9_B9/RConn2 -- TR3_3_9/RConn2
  BRK_L3-9_B9/RConn3 -- TR3_3_9/RConn3
  VI_Bus9/LConn1 -- BRK_L3-9_B9/LConn1
  VI_Bus9/LConn2 -- BRK_L3-9_B9/LConn2
  VI_Bus9/LConn3 -- BRK_L3-9_B9/LConn3
  BRK_L2-7_B7/RConn1 -- TR2_2_7/RConn1
  BRK_L4-5_B4/RConn1 -- L4-5/LConn1
